simulink subsystem "controller_skeleton"  (R2023b)
settings: Solver=VariableStepAuto  StartTime=0.0  StopTime=10.0  RelTol=1e-3
undefined symbols (not defined in the file or in its folder): sim
settings Model: Creator=Inver  LastModifiedBy=TAK

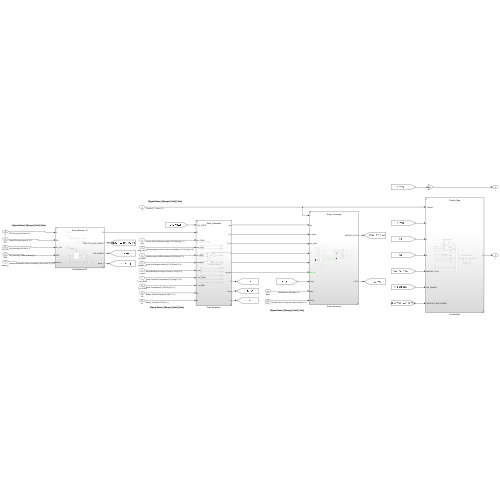
[thumbnail: Simulink's stored preview of the top-level diagram]
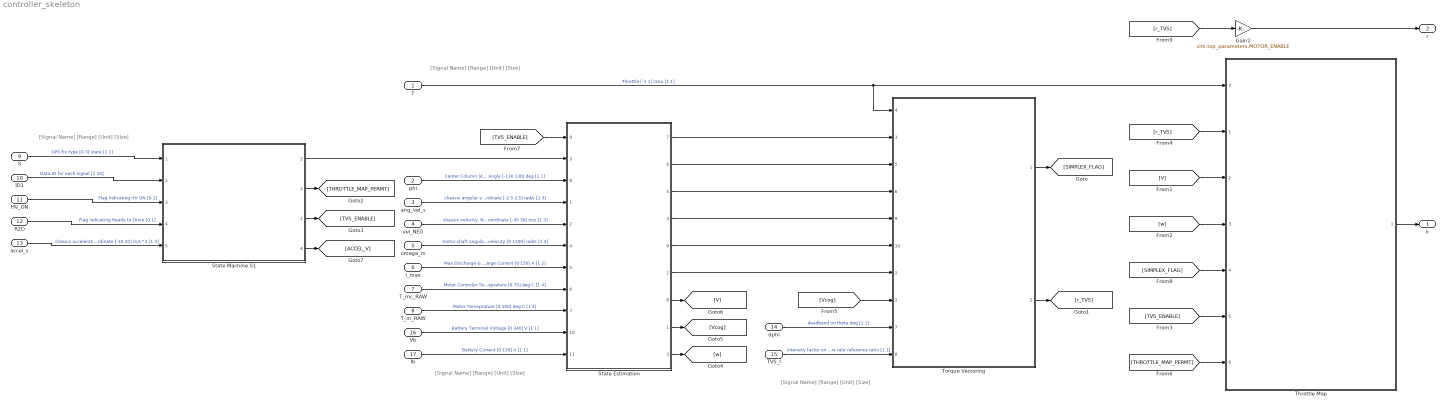
== system controller_skeleton ==
  note: [Signal Name] [Range] [Unit] [Size]
  note: [Signal Name] [Range] [Unit] [Size]
  note: [Signal Name] [Range] [Unit] [Size]
  note: [Signal Name] [Range] [Unit] [Size]
  T : Inport
  phi : Inport  Port=2
  ang_vel_s : Inport  Port=3
  vel_NED : Inport  Port=4
  omega_m : Inport  Port=5
  i_max : Inport  Port=6
  T_mc_RAW : Inport  Port=7
  T_m_RAW : Inport  Port=8
  S : Inport  Port=9
  ID1 : Inport  Port=10
  HV_ON : Inport  Port=11
  R2D : Inport  Port=12
  accel_s : Inport  Port=13
  dphi : Inport  Port=14
  TVS_I : Inport  Port=15
  Vb : Inport  Port=16
  Ib : Inport  Port=17
  Gain2 : Gain  Gain=sim.top_parameters.MOTOR_ENABLE
  State Estimation : Subsystem  ReferencedSubsystem=State_Estimation
      settings: PortSchema="{\"entries\":[{\"content\":{\"sides\":[{\"content\":{\"connectorIds\":[\"In9\",\"In3\",\"In8\",\"In1\",\"In2\",\"In4\",\"In5\",\"In6\",\"In7\",\"In10\",\"In11\"]},\"type\":\"ConnectorPlacement.EquallySpacedRectSide\",\"uuid\":\"a788c4af-c868-4742-81ae-137d8550b7dd\"},{\"content\":{\"connectorIds\":[\"Out7\",\"Out6\",\"Out5\",\"Out4\",\"Out9\",\"Out2\",\"Out8\",\"Out1\",\"Out3\"],\"side\":\"RIGHT\"},\"type\":\"ConnectorPlacement.EquallySpacedRectSide\",\"uuid\":\"40c1d3ed-7f96-4f50-8201-1fa73cbd293c\"},{\"content\":{\"side\":\"TOP\"},\"type\":\"ConnectorPlacement.EquallySpacedRectSide\",\"uuid\":\"412486a9-9897-40de-926c-efa6067c47b5\"}]},\"type\":\"ConnectorPlacement.EquallySpacedConnector\",\"uuid\":\"e2349428-ea4b-4d6c-9a0f-70e14711b204\"}],\"packageUris\":[\"http://schema.mathworks.com/mf0/Connector/R2020b\"],\"version\":\"1.0\"}"
  State Machine S1 : Subsystem  ReferencedSubsystem=State_Machine_S1
      settings: PortSchema="{\"entries\":[{\"content\":{\"sides\":[{\"content\":{\"connectorIds\":[\"In1\",\"In2\",\"In3\",\"In4\",\"In5\"]},\"type\":\"ConnectorPlacement.EquallySpacedRectSide\",\"uuid\":\"0ceeb5ea-6d0e-4b11-9c77-4c2d2629aa1d\"},{\"content\":{\"connectorIds\":[\"Out2\",\"Out3\",\"Out1\",\"Out4\"],\"side\":\"RIGHT\"},\"type\":\"ConnectorPlacement.EquallySpacedRectSide\",\"uuid\":\"93ae308c-ab06-4805-a14d-b44312a3e2f5\"},{\"content\":{\"side\":\"TOP\"},\"type\":\"ConnectorPlacement.EquallySpacedRectSide\",\"uuid\":\"a6b069bc-7653-4744-801e-ae6b7d98ca72\"}]},\"type\":\"ConnectorPlacement.EquallySpacedConnector\",\"uuid\":\"66695feb-77ec-47e7-a8ac-84b2b4d94795\"}],\"packageUris\":[\"http://schema.mathworks.com/mf0/Connector/R2020b\"],\"version\":\"1.0\"}"
  Throttle Map : Subsystem  ReferencedSubsystem=Throttle_Map
      settings: PortSchema="{\"entries\":[{\"content\":{\"sides\":[{\"content\":{\"connectorIds\":[\"In7\",\"In1\",\"In2\",\"In3\",\"In4\",\"In5\",\"In6\"]},\"type\":\"ConnectorPlacement.EquallySpacedRectSide\",\"uuid\":\"0a2325a3-9d51-4087-b02d-3e382446227a\"},{\"content\":{\"connectorIds\":[\"Out1\"],\"side\":\"RIGHT\"},\"type\":\"ConnectorPlacement.EquallySpacedRectSide\",\"uuid\":\"1dae26bb-0e0b-4c8e-9d40-43caeaa44005\"},{\"content\":{\"side\":\"TOP\"},\"type\":\"ConnectorPlacement.EquallySpacedRectSide\",\"uuid\":\"12710057-5a58-45a8-acf5-4b6ffc7139ef\"}]},\"type\":\"ConnectorPlacement.EquallySpacedConnector\",\"uuid\":\"fad868a8-f7f5-4d78-95c0-434c459d05fc\"}],\"packageUris\":[\"http://schema.mathworks.com/mf0/Connector/R2020b\"],\"version\":\"1.0\"}"
  Torque Vectoring : Subsystem  ReferencedSubsystem=Torque_Vectoring
      settings: PortSchema="{\"entries\":[{\"content\":{\"sides\":[{\"content\":{\"connectorIds\":[\"In4\",\"In3\",\"In5\",\"In6\",\"In9\",\"In10\",\"In2\",\"In1\",\"In7\",\"In8\"]},\"type\":\"ConnectorPlacement.EquallySpacedRectSide\",\"uuid\":\"e5337710-7afc-44d5-961b-efcd80b22325\"},{\"content\":{\"connectorIds\":[\"Out1\",\"Out2\"],\"side\":\"RIGHT\"},\"type\":\"ConnectorPlacement.EquallySpacedRectSide\",\"uuid\":\"7e97e5bc-3983-40c2-bdf4-f229f862f80b\"},{\"content\":{\"side\":\"TOP\"},\"type\":\"ConnectorPlacement.EquallySpacedRectSide\",\"uuid\":\"1eebe57d-188b-4569-998a-307371d30e4f\"}]},\"type\":\"ConnectorPlacement.EquallySpacedConnector\",\"uuid\":\"25a81eaa-afe2-4445-a3db-4a69d15d4e62\"}],\"packageUris\":[\"http://schema.mathworks.com/mf0/Connector/R2020b\"],\"version\":\"1.0\"}"
  k : Outport
  r : Outport  Port=2
  wires:
  T/1 -> Torque Vectoring/4, Throttle Map/7  "Throttle [-1 1] ratio [1 1]"
  phi/1 -> State Estimation/8  "Center Column Steering Angle [-130 130] deg [1 1]"
  ang_vel_s/1 -> State Estimation/1  "chassis angular velocity, sensor coordinate [-2.5 2.5] rad/s [1 3]"
  vel_NED/1 -> State Estimation/2  "chassis velocity, NED coordinate [-30 30] m/s [1 3]"
  omega_m/1 -> State Estimation/4  "motor shaft angular velocity [0 1100] rad/s [1 4]"
  i_max/1 -> State Estimation/5  "Max Discharge & Charge Current [0 150] A [1 2]"
  T_mc_RAW/1 -> State Estimation/6  "Motor Controler Temeprature [0 75] deg C [1 4]"
  T_m_RAW/1 -> State Estimation/7  "Motor Temeprature [0 100] deg C [1 4]"
  S/1 -> State Machine S1/1  "GPS fix type [0 3] state [1 1]"
  ID1/1 -> State Machine S1/2  "Data ID for each signal [1 10]"
  Throttle Map/1 -> k/1
  [V] -> Throttle Map/2
  [w] -> Throttle Map/3
  [TVS_ENABLE] -> Throttle Map/5
  dphi/1 -> Torque Vectoring/7  "deadband on theta deg [1 1]"
  TVS_I/1 -> Torque Vectoring/8  "intensity factor on yaw rate reference ratio [1 1]"
  State Estimation/2 -> Torque Vectoring/2
  Torque Vectoring/1 -> [SIMPLEX_FLAG]
  [SIMPLEX_FLAG] -> Throttle Map/4
  HV_ON/1 -> State Machine S1/3  "Flag Indicating HV ON [0 1]"
  R2D/1 -> State Machine S1/4  "Flag Indicating Ready to Drive [0 1]"
  accel_s/1 -> State Machine S1/5  "chassis acceleration sensor coordinate [-20 20] m/s^2 [1 3]"
  State Machine S1/3 -> [THROTTLE_MAP_PERMT]
  State Machine S1/1 -> [TVS_ENABLE]
  State Machine S1/2 -> State Estimation/3
  [TVS_ENABLE] -> State Estimation/9
  State Estimation/7 -> Torque Vectoring/3
  State Estimation/6 -> Torque Vectoring/5
  State Estimation/5 -> Torque Vectoring/6
  State Estimation/4 -> Torque Vectoring/9
  State Estimation/3 -> [w]
  State Estimation/1 -> [Vcog]
  [Vcog] -> Torque Vectoring/1
  Vb/1 -> State Estimation/10  "Battery Terminal Voltage [0 340] V [1 1]"
  State Estimation/8 -> [V]
  Ib/1 -> State Estimation/11  "Battery Current [0 150] A [1 1]"
  State Estimation/9 -> Torque Vectoring/10
  Gain2/1 -> r/1
  [THROTTLE_MAP_PERMT] -> Throttle Map/6
  Torque Vectoring/2 -> [r_TVS]
  [r_TVS] -> Throttle Map/1
  [r_TVS] -> Gain2/1
  State Machine S1/4 -> [ACCEL_V]
